simulink model "DC_grid_SCPF"  (R2023b)
settings: Solver=FixedStepAuto  StartTime=0.0  StopTime=5  FixedStep=ts  RelTol=1e-3
values from neighbouring files (symbols this model uses):
  C = 1.4e-3    (= 0.0014)    [param.m]
  Ic = 300    [param.m]
  L = 0.6e-3    (= 0.0006)    [param.m]
  Lt = 100    [param.m]
  nt = Essaim(1,index)    [ObjContr.m]    (also in param.m = 5)
  Ps_ref = 2.5e6    (= 2500000)    [param.m]
  R = 40e-3    (= 0.04)    [param.m]
  Rsh = 50e-3    (= 0.05)    [param.m]
  ts = 1e-4    (= 0.0001)    [param.m]
  Ve = 5e3    (= 5000)    [param.m]
libraries: spsCurrentMeasurementLib x3, spsSeriesRLCBranchLib x3, spsVoltageMeasurementLib x2, spsControlledCurrentSourceLib x1, spsDCVoltageSourceLib x1, spsGroundLib x1, spsControlledVoltageSourceLib x1, sps_lib x1
settings Model: Creator=user  LastModifiedBy=metta
settings DebuggingCC: AlgebraicLoopMsg=none

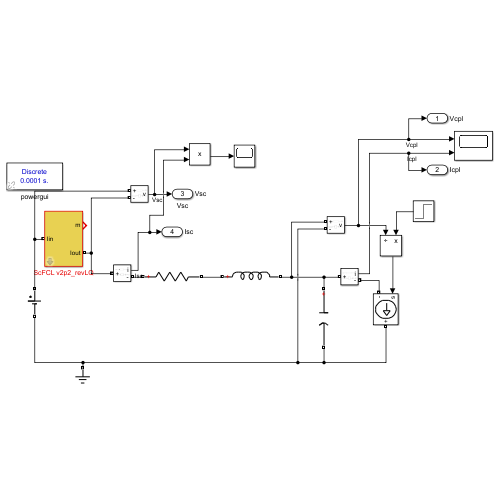
[thumbnail: Simulink's stored preview of the top-level diagram]
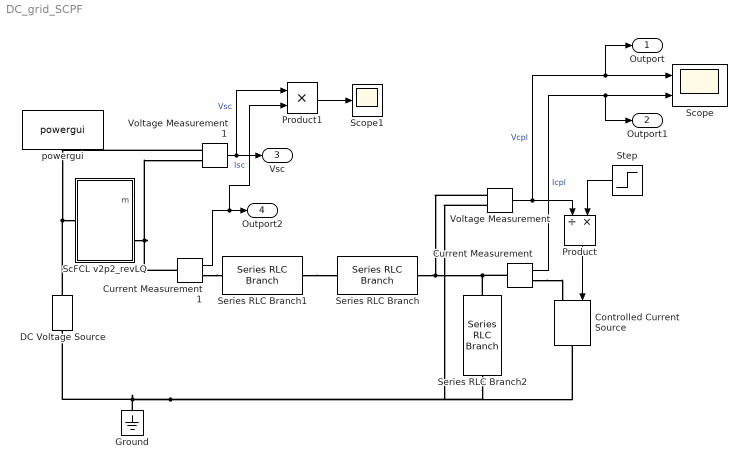
== system DC_grid_SCPF ==
  Controlled Current Source : spsControlledCurrentSourceLib/Controlled Current Source  Initialize=on  Source_Type=DC  Amplitude=0  Phase=0  Frequency=0  Measurements=None
  Current Measurement : spsCurrentMeasurementLib/Current Measurement  PhasorSimulation=off  OutputType=Complex  PSBequivalent=0
  Current Measurement1 : spsCurrentMeasurementLib/Current Measurement  PhasorSimulation=off  OutputType=Complex  PSBequivalent=0
  DC Voltage Source : spsDCVoltageSourceLib/DC Voltage Source  Amplitude=Ve  Measurements=None
  Ground : spsGroundLib/Ground  LConnTagsString=a
  Product : Product  Inputs=/*
  Product1 : Product  Inputs=**
  ScFCL v2p2_revLQ : Subsystem  mask{isScFCLWanted=on, isYBCOWanted=YBCO, Tc_ybco=92, Ic0_ybco=Ic, n0_ybco=21, tw_ybco=12, splicelessTapeLength=Lt, th_ins_ybco=32, th_stab_t=20, th_Ag_t=4, th_Sc=1, th_Hast=100, th_Ag_b=1, th_stab_b=20, Tc_bscco=110, Ic0_bscco=220, n0_bscco=15, tw_bscco=4, fSc_bscco=65, th_ins_bscco=32, th_stab_bscco=0, th_Agbscco=200, RSh=Rsh, tl=Lt, nt=nt, Tref=77, isConvectionWanted=LN2 convection curve  1}
      mask prompts: isScFCLWanted "Enable/Disable ScFCL"; isYBCOWanted "Choice of Material"; Tc_ybco "Critical temperature [K]"; Ic0_ybco "Critical current at 77 K, SF [A]"; n0_ybco "n-value at 77 K, SF"; tw_ybco "Tape width [mm]"; splicelessTapeLength "Spliceless length of tape [m]"; th_ins_ybco "Insulation"; th_stab_t "Stabilizer top"; th_Ag_t "Silver top"; th_Sc "Superconductor"; th_Hast "Hastelloy"; th_Ag_b "Silver bottom"; th_stab_b "Stabilizer bottom"; Tc_bscco "Critical temperature [K]"; Ic0_bscco "Critical current at 77 K, SF [A]"; n0_bscco "n-value at 77 K, SF"; tw_bscco "Tape width [mm]"; fSc_bscco "Percentage of superconductor"; th_ins_bscco "Insulation"; th_stab_bscco "Additional stabilizer (Cu, 304SS, ...)"; th_Agbscco "Ag-BSCCO"; RSh "Shunt resistance [Ohm]:"; tl "Length of tapes [m]:"; nt "Number of tapes in parallel"; Tref "Temperature of reference [K]"; isConvectionWanted "Cooling scheme"
      mask init:
      | if ~isScFCLWanted
      |     tl = 1e-24;
      | end
      | switch isYBCOWanted
      |     case 1 %YBCO
      |         Tc = Tc_ybco;
      |         Ic0 = Ic0_ybco;
      |         n0 = n0_ybco;
      |         tw = 1e-3*tw_ybco; %[m]
      |         th = 1e-6*[th_ins_ybco; th_stab_t; th_Ag_t; th_Sc; th_Hast; th_Ag_b; th_stab_b; th_ins_ybco]; %[m]
      |         th(th == 0) = 1e-12; % If some thickness are zeros, replace by a small value to allow a proper conditioning of the matrix of the system
      |         frac_sc = 0; % not used
      |         % Splice resistivity = ~40 nOhm-cm^2, 10 cm long splice according to:
      |         % Y. Tsui1, E. Surrey and D. Hampshire, "Soldered joints—an essential component of
      |         % demountable high temperature SC fusion magnets," Supercond. Sci. Technol. 29 (2016) 075005 (16pp).
      |         %Rj = (40e-9/(10*tw*1e-2))*ceil(tl/splicelessTapeLength);
      |         Rj = (1e-9)*ceil(tl/splicelessTapeLength);
      |         % It is important to provide a small resistance Rj to Rsc to avoid a bad
      |         % conditioning of the problem (RCOND = Nan in Matlab). It is less
      |         % articifial and more realistic than affecting an arbitrary value to Rsc.
      |     case 2 %BSCCO
      |         Tc = Tc_bscco;
      |         Ic0 = Ic0_bscco;
      |         n0 = n0_bscco;
      |         tw = 1e-3*tw_bscco;
      |         th = 1e-6*[th_ins_bscco; th_stab_bscco/2; th_Agbscco; th_stab_bscco/2; th_ins_bscco; 0; 0; 0]; % artificially increase the dimension for allowing persistent values and switching between materials
      |         th(th == 0) = 1e-12; 
      |         frac_sc = fSc_bscco/100; % prercentage
      |         Rj = 20e-9;
      |     otherwise % Do nothing yet
      |         Tc = Tc_ybco;
      |         Ic0 = Ic0_ybco;
      |         n0 = n0_ybco;
      |         tw = 1e-3*tw_ybco; %[m]
      |         th = 1e-6*[th_ins_ybco; th_stab_t; th_Ag_t; th_Sc; th_Hast; th_Ag_b; th_stab_b; th_ins_ybco]; %[m]
      |         th(th == 0) = 1e-12; % If some thickness are zeros, replace by a small value to allow a proper conditioning of the matrix of the system
      |         frac_sc = 0; % not used
      |         Rj = 20e-9;
      | end
      mask TypeOptions isYBCOWanted: YBCO | BSCCO
      mask TypeOptions isConvectionWanted: No thermal model (T=Tref) | Adiabatic | LN2 convection curve  1 | LN2 convection curve 2 | LN2 convection curve 3
      mask DialogControl MaterialContainer Prompt: Material properties
      mask DialogControl YBCOContainer Prompt: YBCO
      mask DialogControl ThicknessesYBCOContainer Prompt: Thickness of tape layers [um]
      mask DialogControl BSCCOContainer Prompt: BSCCO
      mask DialogControl ThicknessesBSCCOContainer Prompt: Thickness of tape layers [um]
      mask DialogControl ScFCLContainer Prompt: ScFCL
      mask DialogControl CoolingContainer Prompt: Cooling options
  Scope : Scope  NumInputPorts=2
  Scope1 : Scope
  Series RLC Branch : spsSeriesRLCBranchLib/Series RLC Branch  LConnTagsString=__new0  RConnTagsString=__new0  BranchType=L  Resistance=R  Inductance=L  SetiL0=off  InitialCurrent=0  Capacitance=1e-6  Setx0=off  InitialVoltage=0  Measurements=None
  Series RLC Branch1 : spsSeriesRLCBranchLib/Series RLC Branch  LConnTagsString=__new0  RConnTagsString=__new0  BranchType=R  Resistance=R  Inductance=1e-3  SetiL0=off  InitialCurrent=0  Capacitance=1e-6  Setx0=off  InitialVoltage=0  Measurements=None
  Series RLC Branch2 : spsSeriesRLCBranchLib/Series RLC Branch  LConnTagsString=__new0  RConnTagsString=__new0  BranchType=C  Resistance=R  Inductance=L  SetiL0=off  InitialCurrent=0  Capacitance=C  Setx0=off  InitialVoltage=0  Measurements=None
  Step : Step  Time=0.1  After=Ps_ref  SampleTime=0
  Voltage Measurement : spsVoltageMeasurementLib/Voltage Measurement  PhasorSimulation=off  OutputType=Complex  PSBequivalent=0
  Voltage Measurement1 : spsVoltageMeasurementLib/Voltage Measurement  PhasorSimulation=off  OutputType=Complex  PSBequivalent=0
  powergui : sps_lib/powergui  Priority=1  SimulationMode=Discrete  SampleTime=ts  frequency=60  Iterations=50  frequencyindice=0  Pbase=100e6  ErrMax=1e-4  UnitsV=kV  UnitsW=MW  buscounter=0  FunctionMessages=off  echomessages=off  EnableUseOfTLC=off  CurrentSourceSwitches=off  DisableSnubberDevices=off  DisableRonSwitches=off  DisableVfSwitches=off  DisplayEquations=off  AutomaticDiscreteSolvers=off  SolverType=Tustin/Backward Euler (TBE)  Interpol=off  ExternalGateDelay=off  methode=off  Ts=100  x0status=blocks  SPID=on  SwTol=0  HookPort=off  NonlinearTolerance=1e-4  nMaxIteration=100  ContinueOnMaxIteration=off  RestoreLinks=warning  ResistiveCurrentMeasurement=off  Frange=[0:2:500]  Ylog=off  Xlog=on  ShowGrid=off  save=off  variable=ZData  structure=0  ZoomFFT=off  StartTime=0.0  cycles=1  DisplayStyle=1  fundamental=60  FreqAxis=off  MaxFrequency=1000  frequencyindicesteady=1  RmsSteady=1  display=off
  Outport : Outport  SignalName=Vcpl
  Outport1 : Outport  Port=2  SignalName=Icpl
  Vsc : Outport  Port=3  SignalName=Vsc
  Outport2 : Outport  Port=4  SignalName=Isc
  wires:
  Product/1 -> Controlled Current Source/1
  Current Measurement/1 -> Outport1/1, Scope/2  "Icpl"
  Step/1 -> Product/2
  Voltage Measurement/1 -> Product/1, Outport/1, Scope/1  "Vcpl"
  Voltage Measurement1/1 -> Product1/1, Vsc/1  "Vsc"
  Current Measurement1/1 -> Product1/2, Outport2/1  "Isc"
  Product1/1 -> Scope1/1
  connections:
  Series RLC Branch1/RConn1 -- Series RLC Branch/LConn1
  Series RLC Branch/RConn1 -- Series RLC Branch2/LConn1 -- Current Measurement/LConn1 -- Voltage Measurement/LConn1
  Ground/LConn1 -- Series RLC Branch2/RConn1 -- Controlled Current Source/RConn1 -- Voltage Measurement/LConn2 -- DC Voltage Source/LConn1
  Current Measurement/RConn1 -- Controlled Current Source/LConn1
  DC Voltage Source/RConn1 -- Voltage Measurement1/LConn1 -- ScFCL v2p2_revLQ/LConn1
  ScFCL v2p2_revLQ/RConn1 -- Current Measurement1/LConn1 -- Voltage Measurement1/LConn2
  Current Measurement1/RConn1 -- Series RLC Branch1/LConn1

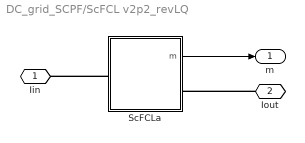
== system DC_grid_SCPF/ScFCL v2p2_revLQ ==
  ScFCLa : Subsystem
  Iin : PMIOPort  Side=Left
  Iout : PMIOPort  Port=2  Side=Right
  m : Outport
  wires:
  ScFCLa/1(m) -> m/1
  connections:
  Iout/RConn1 -- ScFCLa/RConn1
  ScFCLa/LConn1 -- Iin/RConn1

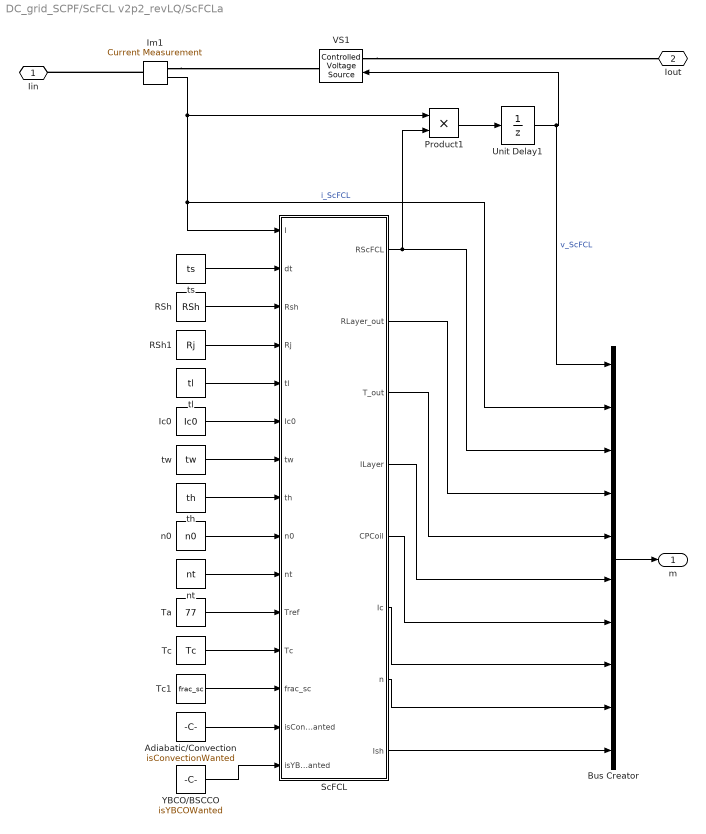
== system DC_grid_SCPF/ScFCL v2p2_revLQ/ScFCLa ==
  Adiabatic/Convection : Constant  Value=isConvectionWanted
  Bus Creator : BusCreator  Inputs=10
  Ic0 : Constant  Value=Ic0
  Im1 : spsCurrentMeasurementLib/Current Measurement  PhasorSimulation=off  OutputType=Complex  PSBequivalent=0
  Product1 : Product
  RSh : Constant  Value=RSh
  RSh1 : Constant  Value=Rj
  ScFCL : MATLAB Function  TreatAsAtomicUnit=on
  Ta : Constant  Value=77
  Tc : Constant  Value=Tc
  Tc1 : Constant  Value=frac_sc
  Unit Delay1 : UnitDelay  SampleTime=ts  HasFrameUpgradeWarning=on
  VS1 : spsControlledVoltageSourceLib/Controlled Voltage Source  Initialize=on  Source_Type=AC  Amplitude=1e-12  Phase=0  Frequency=60  Measurements=None
  YBCO/BSCCO : Constant  Value=isYBCOWanted
  n0 : Constant  Value=n0
  nt : Constant  Value=nt
  th : Constant  Value=th
  tl : Constant  Value=tl
  ts : Constant  Value=ts
  tw : Constant  Value=tw
  Iin : PMIOPort  Side=Left
  Iout : PMIOPort  Port=2  Side=Right
  m : Outport
  wires:
  Adiabatic/Convection/1 -> ScFCL/14(isConvectionWanted)
  ScFCL/1(RScFCL) -> Product1/2, Bus Creator/3
  ScFCL/2(RLayer_out) -> Bus Creator/4
  ScFCL/3(T_out) -> Bus Creator/5
  ScFCL/4(ILayer) -> Bus Creator/6
  ScFCL/5(CPCoil) -> Bus Creator/7
  ScFCL/6(Ic) -> Bus Creator/8
  ScFCL/7(n) -> Bus Creator/9
  nt/1 -> ScFCL/10(nt)
  Ta/1 -> ScFCL/11(Tref)
  n0/1 -> ScFCL/9(n0)
  th/1 -> ScFCL/8(th)
  Tc/1 -> ScFCL/12(Tc)
  Bus Creator/1 -> m/1
  Unit Delay1/1 -> Bus Creator/1, VS1/1  "v_ScFCL"
  RSh/1 -> ScFCL/3(Rsh)
  ts/1 -> ScFCL/2(dt)
  tl/1 -> ScFCL/5(tl)
  Im1/1 -> ScFCL/1(I), Bus Creator/2, Product1/1  "i_ScFCL"
  tw/1 -> ScFCL/7(tw)
  Product1/1 -> Unit Delay1/1
  Ic0/1 -> ScFCL/6(Ic0)
  YBCO/BSCCO/1 -> ScFCL/15(isYBCOWanted)
  Tc1/1 -> ScFCL/13(frac_sc)
  RSh1/1 -> ScFCL/4(Rj)
  ScFCL/8(Ish) -> Bus Creator/10
  connections:
  Im1/LConn1 -- Iin/RConn1
  Im1/RConn1 -- VS1/RConn1
  VS1/LConn1 -- Iout/RConn1

== matlab function DC_grid_SCPF/ScFCL v2p2_revLQ/ScFCLa/ScFCL ==
  data: RScFCL output; I input; RLayer_out output; T_out output; ILayer output; dt input; Rsh input; Rj input; tl input; CPCoil output; Ic0 input; Ic output; tw input; th input; n0 input; nt input; Tref input; Tc input; frac_sc input; n output; isConvectionWanted input; isYBCOWanted input; Ish output
%%% MAIN %%%
%%% Based on Jose Juan Chavez Perez's first model. Modified by Frederic Trillaud <ftrillaudp@gmail.com> & Loic Queval <loic.queval@gmail.com>.
%%% Version: 2.3 20170910
function [RScFCL, RLayer_out, T_out, ILayer, CPCoil, Ic, n, Ish] = ...
    fcn(I, dt, Rsh, Rj, tl, Ic0, tw, th, n0, nt, Tref, Tc, frac_sc, isConvectionWanted, isYBCOWanted)

%% INPUTS
% I ScFCL current [A]
% dt time step [s]
% Rsh shunt resistance [Ohm]
% Rj residual resistance due to joints (splices and connections) plus the AC base dissipation (it is useful to prevent as well a division by zero in the code) [Ohm]
% tl length of tapes [m]
% Ic0 tape critical current at 77 K, SF [A]
% tw tape width [m]
% th vector of layer thickness [m]
% n0 n-value at 77 K, SF []
% nt number of tapes in parallel []
% Tref temperature of reference [K]
% Tc critical temperature at 77 K, SF [K]
% frac_sc ? [?]
% isConvectionWanted: 1=no thermal model, 2=adiabatic, 3=curve 1, 4=curve 2, 5=curve 3 (curves of convection with LN2)
% isYBCOWanted: 1=YBCO, 2=BSCCO, 3=MgB2 unavailable

% To eliminate a layer, enter 0 in the corresponding thickness in the mask
% of the ScFCL simulink model. Automatically, instead of 0, 1e-9 will be used.
% It is necessary to allow a proper conditioning of the matrix system to solve the temperature.

%% OUPUTS
% RScFCL equivalent resistance (equivalent resistance of the fault-current limiter appearing as a resitance for the electrical circuit) [Ohm]
% RLayer_out =  Rlayer resistance of each layer [Ohm]
% T_out = T temperature of each layer [K]
% ILayer current flowing through the each layer [A]
% CPCoil Cooling power exchanged with LN2 for the nt tapes (accumulated exchanged power for the entire set of parallel superconducting tapes to be compred to DPCoil) [W]
% Ic critical current at T, SF [A]
% n n-value at T, SF []

% To do list:
% 1. Change some of the function of thermal properties: 304SS, Cu and Ag for instance to NIST functions
% 2. Add the model of the MgB2

%% Some variables
Swl = tw*tl; % Flat surface of the tape: tape width * tape length [m^2]
Shw = tw*th; % Cross-section of the tape layer [m^2]

%% Initialization
% Inputs from previous time iterations carried out in Simulink
persistent T; %temperature of each layer [K]
persistent RLayer; %resistance of each layer [Ohm]

if isempty(T)
    T = Tref*ones(length(th), 1); %initially the temperature of each layer is Tref
end
if isempty(RLayer)
    RLayer = 1e38*ones(length(th), 1); %initially the resistance of each layer is infinite
end

switch isYBCOWanted
    case 1 % YBCO
        % (1) = top insulation
        % (2) = top stabilizer
        % (3) = top silver
        % (4) = YBCO
        % (5) = Hastelloy
        % (6) = bottom silver
        % (7) = bottom stabilizer
        % (8) = bottom insulation
        
        %%% Update %%%
        
        Ic = IcVersusT(Ic0, T(4), Tc, Tref, isYBCOWanted); % [A] Critical current of the SC layer
        n = nVersusT(n0, T(4), Tref); % [] power law index
        
        %%% Current sharing %%%
        
        % Update the resistance of each layer, RLayer is a persistant variable from the previous step
        %RLayer = Resistance(T, RLayer(4)*(th(4)*tw)/tl, tl, Shw, frac_sc, isYBCOWanted); % [Ohm] Resistance of the various layers (but not the SC layer)
        RLayer = Resistance_2p3(RLayer, T, tl, Shw, frac_sc, isYBCOWanted);
        RLayer(4) = ScResistance(RLayer, Rsh, Rj, I, T(4), Ic, nt, tw, tl, th(4), n, Tc, isYBCOWanted); % [Ohm] Resistance of the SC layer
        
        % Get the current in each layer
        RScFCL = 1/(sum(nt./RLayer)+1/Rsh); % [Ohm] Equivalent resitance of the fault current limiter
        ILayer = (RScFCL./RLayer)*I; % [A] current circulating per layer
        Ish = (RScFCL/Rsh)*I; % [A] shuunt current
        
        %%% Thermal model %%%
        
        DPLayer = RLayer.*ILayer.^2; %[W] dissipated power (DP) per layer
        
        % Cooling power (CP)
        switch isConvectionWanted
            case 2 % Adiabatic
                phi = 0; % heat flux
            case 3 % LN2 convection curve 1
                [HH, phi] = HeatTransfer_1(T(1), Tref); % top
                [HH, phi] = HeatTransfer_1(T(8), Tref); % bottom
            case 4 % LN2 convection curve 2
                [HH, phi] = HeatTransfer_2(T(1), Tref);
                [HH, phi] = HeatTransfer_2(T(8), Tref);
            case 5 % LN2 convection curve 3
                [HH, phi] = HeatTransfer_3(T(1), Tref);
                [HH, phi] = HeatTransfer_3(T(8), Tref);
            otherwise % Infinite reservoir
                phi = inf;
        end
        
        % Estimation of the new temperature:
        if isConvectionWanted ~= 1 %update only if thermal model activated
            T = UpdatedTemperature(T, Swl, th, dt, DPLayer, Tref, frac_sc, isConvectionWanted, isYBCOWanted);
        end
        
    case 2 % BSCCO
        % (1) = top insulation
        % (2) = top stabilizer
        % (3) = Ag matrix
        % (4) = BSCCO
        % (5) = bottom stabilizer,
        % (6) = bottom insulation
        
        %%% Update %%%
        
        Ic = IcVersusT(Ic0, T(3), Tc, Tref, isYBCOWanted); % [A] Critical current of the SC layer
        n = nVersusT(n0, T(3), Tref); % [] power law index
        
        %%% Current sharing %%%
        
        % Update the resistance of each layer, RLayer is a persistant variable from the previous step
        %RLayer = Resistance(T, RLayer(4)*(frac_sc*th(3)*tw)/tl, tl, Shw, frac_sc, isYBCOWanted); % To be consistent with YBCO for future simplification. See the masking function for the definition of th for both YBCO and BSCCO
        RLayer = Resistance_2p3(RLayer, T, tl, Shw, frac_sc, isYBCOWanted);
        RLayer(4) = ScResistance(RLayer, Rsh, Rj, I, T(4), Ic, nt, tw, tl, th(4), n, Tc, isYBCOWanted); % [Ohm] Resistance of the SC layer
        
        % Get the current in each layer
        RScFCL = 1/(sum(nt./RLayer)+1/Rsh); % [Ohm] Equivalent resitance of the fault current limiter
        ILayer = (RScFCL./RLayer)*I; % [A] current circulating per layer
        Ish = (RScFCL/Rsh)*I; % [A] shuunt current
        
        %%% Thermal model %%%
        
        DPLayer = RLayer.*ILayer.^2; %[W] dissipated power (DP) per layer
        DPLayer(1) = DPLayer(1); % Insulation
        DPLayer(2) = DPLayer(2); % Stabilizer
        DPLayer(3) = DPLayer(3)+DPLayer(4);   % Sum of power dissipated by Ag and BSCCO
        DPLayer(4) = DPLayer(5); % stabilizer
        DPLayer(5) = DPLayer(6); % Insulation
        DPLayer(6) = DPLayer(7);
        DPLayer(7) = 0;
        DPLayer(8) = 0;
        
        % Cooling power (CP)
        switch isConvectionWanted
            case 2 % Adiabatic
                phi = 0; % heat flux
            case 3 % LN2 convection curve 1
                [HH, phi] = HeatTransfer_1(T(1), Tref); % top
                [HH, phi] = HeatTransfer_1(T(5), Tref); % bottom
            case 4 % LN2 convection curve 2
                [HH, phi] = HeatTransfer_2(T(1), Tref);
                [HH, phi] = HeatTransfer_2(T(5), Tref);
            case 5 % LN2 convection curve 3
                [HH, phi] = HeatTransfer_3(T(1), Tref);
                [HH, phi] = HeatTransfer_3(T(5), Tref);
            otherwise % Infinite reservoir
                phi = inf;
        end
        
        % Estimation of the new temperature
        if isConvectionWanted ~= 1 %update only if thermal model activated
            T = UpdatedTemperature(T, Swl, th, dt, DPLayer, Tref, frac_sc, isConvectionWanted, isYBCOWanted);
        end
        
    otherwise
        disp('MgB2 to be implemnted');
        
        %%% Update %%%
        
        Ic = 0; % [A] Critical current of the SC layer
        n = 0; % [] power law index
        
        %%% Current sharing %%%
        
        RScFCL = inf; % [Ohm] Equivalent resitance of the fault current limiter
        ILayer = zeros(length(th), 1); % [A] current circulating per layer
        Ish = 0; % [A] shuunt current
        
        %%% Thermal model %%%
        
        DPLayer = ones(length(th), 1); %[W] dissipated power (DP) per layer
        phi = inf;
        
end

CPTapet = Swl*phi;
CPTapeb = Swl*phi;
CPCoil = nt*(CPTapet+CPTapeb); % Cooling power exchanged with LN2 for the nt tapes

% For exiting the function without error and save the current values for the next time step carried out in Simulink
T_out = T;
RLayer_out = RLayer;

end


%% AUXILIARY FUNCTIONS

% Resistance per tape
function value_R = Resistance(T, rho_sc, tl, Shw, frac_sc, isYBCOWanted) % TO DELETE IF OK

switch isYBCOWanted
    case 1 % YBCO
        rho1  = 1e25; % insulation
        rho2  = rho_Cu(T(2));
        rho3  = rho_Ag(T(3));
        rho5  = rho_Hastelloy(T(5));
        rho6  = rho_Ag(T(6));
        rho7  = rho_Cu(T(7));
        rho8  = 1e25; % insulation
        rho   = [rho1; rho2; rho3; rho_sc; rho5; rho6; rho7; rho8]; %[Ohm.m]
        R = (tl*rho)./Shw;
    case 2 % BSCCO
        rho1  = 1e25; % insulation
        rho2  = rho_Cu(T(2));
        rho3 = rho_Ag(T(3))/(1-frac_sc);
        rho5  = rho_Cu(T(4));
        rho6  = 1e25; % insulation
        rho = [rho1; rho2; rho3; rho_sc; rho5; rho6; 0; 0]; %[Ohm.m]
        R1 = (tl*rho1)/Shw(1);
        R2 = (tl*rho2)/Shw(2);
        R3 = (tl*rho3)/((1-frac_sc)*Shw(3));
        R4 = (tl*rho_sc)/(frac_sc*Shw(3));
        R5 = (tl*rho5)/Shw(4);
        R6 = (tl*rho6)/Shw(5);
        % Adding large resistivity to allow a proper computation of the
        % current layers and dissipation to solve the temperature
        R = [R1; R2; R3; R4; R5; R6; 1e38; 1e38];
    otherwise
        disp('MgB2 to be implemnted');
        rho = ones(8, 1);
        R = (tl*rho)./Shw;
end

value_R = R; %[Ohm]

end

% Update resistance of the layers except SC layer
function R = Resistance_2p3(R, T, tl, Shw, frac_sc, isYBCOWanted)

switch isYBCOWanted
    case 1 % YBCO
        %R(1) %[Ohm] top insulation
        R(2)  = rho_Cu(T(2))*tl/Shw(2); %[Ohm] top stabilizer
        R(3)  = rho_Ag(T(3))*tl/Shw(3); %[Ohm] top silver
        %R(4) %[Ohm] YBCO
        R(5)  = rho_Hastelloy(T(5))*tl/Shw(5); %[Ohm] Hastelloy
        R(6)  = rho_Ag(T(6))*tl/Shw(6); %[Ohm] bottom silver
        R(7)  = rho_Cu(T(7))*tl/Shw(7); %[Ohm] bottom stabilizer
        %R(8) %[Ohm] bottom insulation
    case 2 % BSCCO
        %R(1) %[Ohm] top insulation
        R(2) = rho_Cu(T(2))*tl/Shw(2); %[Ohm] top stabilizer
        R(3) = (rho_Ag(T(3))/(1-frac_sc))*tl/((1-frac_sc)*Shw(3)); %[Ohm] Ag matrix
        %R(4) = rho_sc*tl/(frac_sc*Shw(3)); %[Ohm] BSCCO
        R(5) = rho_Cu(T(4))*tl/Shw(4); %[Ohm] bottom stabilizer
        %R(6) %[Ohm] bottom insulation
        %R(7) %[Ohm] empty
        %R(8) %[Ohm] empty
    otherwise
        disp('MgB2 to be implemnted');
end

end

% Resistance of the superconductor [Ohm]
function value_Rsc = ScResistance(Rlayer, Rsh, Rj, I, Tsc, Ic, nt, tw, tl, thsc, n, Tc, isYBCOWanted)
% I = ScFCL current
% Ic = SC layer critical current
% value_Rsc = SC layer resistance in series with Rj

if (Tsc < Tc)
    % Critical electrical field and voltage
    Ec = 1e-4;  % [V/m] (1e-6*100)
    Vc = Ec*tl; % [V]
    
    % Current sharing with Newton algorithm
    RScFCL = 1/(sum(nt./Rlayer)+1/Rsh); % [Ohm] Equivalent resitance of the fault current limiter
    Rsc0 = Rlayer(4)/nt; % [Ohm] Equivalent resitance of all the SC components making the ScFCL
    Rm = 1/(1/Rlayer(2)+1/Rlayer(3)+1/Rlayer(5)+1/Rlayer(6)+1/Rlayer(7)); % [Ohm] Equivalent resitance of all the metallic layers of 1 tape
    Req = Rm*Rsh/(nt*Rsh+Rm); % [Ohm] (Rm/nt)//Rsh
    
    %version 2.2: look for the sum of the currents of the SC layers
    %     ISc0 = (RScFCL/Rsc0)*abs(I); % Aproximation of the target current (absolute value)= sum of SC layers currents
    %     ISc = NewtonRh_2p2(abs(I), ISc0, Vc, n, nt*Ic, Req); % Get sum of SC layers currents, proper than scaling to the resistance. Otherwise, it is assumed that the changing are smooth enough to be caught from the previous time step. I do not think that it is true with a large n-value.
    %     Rsc_1 = (Vc*ISc^(n-1)/((nt*Ic)^n))*nt; % ok because keep in mind that this is Ic*=m*Ic
    
    %version 2.3: look for the current in one SC layer
    ISc0 = (RScFCL/Rsc0)*abs(I)/nt; % Aproximation of the target current (absolute value)= current of the SC layer
    ISc = NewtonRh_2p3(abs(I), ISc0, Vc, n, Ic, Req, nt); % Get current of the SC layer current, proper than scaling to the resistance. Otherwise, it is assumed that the changing are smooth enough to be caught from the previous time step. I do not think that it is true with a large n-value.
    Rsc_1 = (Vc*ISc^(n-1)/(Ic^n));
    
    switch isYBCOWanted
        case 1 % YBCO
            Rsc_2 = rho_YBCO(Tsc)*tl/(thsc*tw);
        case 2 %BSCCO
            Rsc_2 = rho_BSCCO(Tsc, Tc)*tl/(thsc*tw);
        otherwise
            Rsc_2 = rho_YBCO(Tsc)*tl/(thsc*tw);
    end
    Rsc  = min(Rsc_1, Rsc_2);
    
else % Normal state
    switch isYBCOWanted
        case 1 % YBCO
            Rsc = rho_YBCO(Tsc)*tl/(thsc*tw);
        case 2 %BSCCO
            Rsc = rho_BSCCO(Tsc, Tc)*tl/(thsc*tw);
        otherwise
            Rsc = rho_YBCO(Tsc)*tl/(thsc*tw);
    end
end

value_Rsc = Rsc+Rj; % better than putting a condition to ensure a proper conditioning of the system (avoiding division by zero). In addition, it makes sense that there should be a base dissipation and slices driving a residual resistance at the superconducting layer.

end

% Current sharing
function value_ISc = NewtonRh_2p2(I, Isc0, Vc, n, Ic, Req)

%stop conditions
maxIter = 1000;
tol = 1e-6;

%initialization
error = 1000; %initialize the error
j = 1; %initialize the iteration number
Isc = Isc0; %initial guess

while ((error > tol) && (j <= maxIter))
    f = Vc*(Isc/Ic)^n+Req*Isc-Req*I;
    df = n* Vc*Isc^(n-1)/(Ic^n)+Req;
    Isc = Isc-f/df;
    
    error = abs(f);
    j = j+1;
    if (j > maxIter)
        disp('Maximum number of iteration reached, error = %g', error);
        break
    end
end

value_ISc = Isc;

end

function value_ISc = NewtonRh_2p3(I, Isc0, Vc, n, Ic, Req, nt)

%stop conditions
maxIter = 1000;
tol = 1e-6;

%initialization
error = 1000; %initialize the error
j = 1; %initialize the iteration number
Isc = Isc0; %initial guess

while ((error > tol) && (j <= maxIter))
    f = Vc*(Isc/Ic)^n - Req*I + Req*nt*Isc;
    df = n*Vc*Isc^(n-1)/Ic^n + Req*nt;
    Isc = Isc-f/df;
    
    error = abs(f);
    j = j+1;
    if (j > maxIter)
        disp('Maximum number of iteration reached, error = %g', error);
        break
    end
end

value_ISc = Isc;

end

% Ic versus T: For the moment there is no need to change or change it. I
% like to keep a certain generality at least until the version is
% completely frozen. Matter of taste.
function value_Ic = IcVersusT(Ic0, Tsc, Tc, Tref, isYBCOWanted)

switch isYBCOWanted
    case 1 % YBCO
        Ic = Ic0*(Tc-Tsc)/(Tc-Tref);
        % I propose: value_Ic = Ic0*(Tc-Tsc)/(Tc-77);
    case 2 % BSCCO
        TTref = Tsc/Tref; % TTref = Tsc/77;
        a0 = 31.1533948715955;
        a1 = -195.759566845438;
        a2 = 588.409496514242;
        a3 = -930.754142719088;
        a4 = 793.067560549802;
        a5 = -345.73762156648;
        a6 = 60.6210777447419;
        Ic = Ic0*(a0+a1*TTref+a2*TTref^2+a3*TTref^3+a4*TTref^4+a5*TTref^5+a6*TTref^6);
    otherwise
        Ic = Ic0*(Tc-Tsc)/(Tc-Tref);
end

value_Ic = Ic;

end

% N-value versus T: see previous function
function value_n = nVersusT(n0, Tsc, Tref)
value_n = n0*Tref/Tsc;
% I propose: value_n = n0*77/Tsc;
end

% Update the Temperature of the layers from Electro-thermal equivalent:
% (C, G, CG): C(Tnew-Tol)/dt = G(Told)*Tnew+CG(Told)*Tref+Qtold, pseudo-implicit Method;
% In the simulink model ts is equal to dt, ts being the time step
function value_T = UpdatedTemperature(T, Swl, th, dt, Qt, Tref, frac_sc, isConvectionWanted, isYBCOWanted)

% Matrices of heat dissipation and thermal conductances:
C = HeatCapacity(T, Swl, th, frac_sc, isYBCOWanted); % Matrix of heat capacity
G = ThermalConductance(T, Swl, th, Tref, frac_sc, isConvectionWanted, isYBCOWanted); % matrix of thermal conductance per mid layer
CG = ConvectiveConductance(T, Swl, th, Tref, isConvectionWanted, isYBCOWanted); % matrix of thermal conductance at the boundary per tape

T = inv(C+dt*G)*(C*T+dt*(CG*Tref+Qt));
% [LOIC] if you solve C(Tnew-Tol)/dt = G(Told)*Tnew+CG(Told)*Tref+Qtold, then
% G<0 and the implicit method gives:
% I do not understand. See my notes that I sent (thermal model). G is a
% matrix. If you change the sign, you have to revert the sign into the
% definition of G. It is done this way to fit the mathematical model.
% T = inv(C-dt*G)*(C*T+dt*(CG*Tref+Qt));

value_T = T;

end

% Heat capacity [J/K]
function value_C = HeatCapacity(T, Swl, th, frac_sc, isYBCOWanted)
% Density of layer materials (kg/m^3)
Dins = 1420;     % Kapton
DAg = 10470;     % Silver
DYBCO = 6300;    % YBCO
DHast = 8900;    % Hastelloy
DCu = 8960;      % Copper
DBSCCO = 6500;  % BiSCCO
D304SS = 8000;   % 304 SS

switch isYBCOWanted
    case 1 % YBCO
        % Heat capacity per layer
        Cinst = Swl*th(1)*Dins*SpecificHeatCapacity_Kapton(T(1));      % Insulation top
        CCut = Swl*th(2)*DCu*SpecificHeatCapacity_Cu(T(2));            % Stabilizer top
        CAgt = Swl*th(3)*DAg*SpecificHeatCapacity_Ag(T(3));            % Silver top
        CYBCO = Swl*th(4)*DYBCO*SpecificHeatCapacity_YBCO(T(4));       % YBCO
        CHast = Swl*th(5)*DHast*SpecificHeatCapacity_Hastelloy(T(5));  % Hastelloy
        CAgb = Swl*th(6)*DAg*SpecificHeatCapacity_Ag(T(6));            % Silver bottom
        CCub = Swl*th(7)*DCu*SpecificHeatCapacity_Cu(T(7));            % Stabilizer bottom
        Cinsb = Swl*th(8)*Dins*SpecificHeatCapacity_Kapton(T(8));      % Insulation bottom
        C = diag([Cinst, CCut, CAgt, CYBCO, CHast, CAgb, CCub, Cinsb]);  % diagonal matrix of heat capacities
    case 2 % BSCCO
        Cinst = Swl*th(1)*Dins*SpecificHeatCapacity_Kapton(T(1));        % Insulation top
        CStabt = Swl*th(2)*DCu*SpecificHeatCapacity_Cu(T(2));            % Stabilizer top
        CBSCCO = DBSCCO*SpecificHeatCapacity_BSCCO(T(3));                % BSCCO
        CAg = DAg*SpecificHeatCapacity_Ag(T(3));                         % Silver
        CAgBSCCO = ((1-frac_sc)*CAg+frac_sc*CBSCCO)*Swl*th(3);           % Ag-BSCCO
        CStabb = Swl*th(4)*DCu*SpecificHeatCapacity_Cu(T(4));            % Stabilizer bottom
        Cinsb = Swl*th(5)*Dins*SpecificHeatCapacity_Kapton(T(5));      % Insulation bottom
        % adding 1 to get an inversible matrix inv(C+dt*G) = inv(C), det(C) diff 0
        C = diag([Cinst, CStabt, CAgBSCCO, CStabb, Cinsb, 1, 1, 1]);  % diagonal matrix of heat capacities
    otherwise
        disp('MgB2 to be impmented');
        C = ones(8, 1);
end

value_C = C;

end

% Thermal conductance [W/K]
function value_G = ThermalConductance(T, Swl, th, Tref, frac_sc, isConvectionWanted, isYBCOWanted)

% Thermal resisance by convection on LN2 (K/W);
[THRconvt, THRconvb] = ConvectiveThermalResistance(T, Swl, Tref, isConvectionWanted, isYBCOWanted);

switch isYBCOWanted
    case 1 % YBCO
        % Thermal resistance per layer (K/W):
        THRinst = th(1)/(ThermalConductivity_Kapton(T(1))*Swl);     % Insulation top
        THRCut  = th(2)/(ThermalConductivity_Cu(T(2))*Swl);         % Stabilizer top
        THRAgt  = th(3)/(ThermalConductivity_Ag(T(3))*Swl);         % Silver top
        THRYBCO = th(4)/(ThermalConductivity_YBCO(T(4))*Swl);       % YBCO
        THRHast = th(5)/(ThermalConductivity_Hastelloy(T(5))*Swl);  % Hastelloy
        THRAgb  = th(6)/(ThermalConductivity_Ag(T(6))*Swl);         % Silver bottom
        THRCub  = th(7)/(ThermalConductivity_Cu(T(7))*Swl);         % Stabilizer bottom
        THRinsb = th(8)/(ThermalConductivity_Kapton(T(8))*Swl);     % Insulation bottom
        
        % Thermal conductivity of the different mid layers (see thermal-electric analogy)
        G01 = 1/(THRconvt+THRinst/2);
        G12 = 1/(THRinst/2+THRCut/2);
        G23 = 1/(THRCut/2+THRAgt/2);
        G34 = 1/(THRAgt/2+THRYBCO/2);
        G45 = 1/(THRYBCO/2+THRHast/2);
        G56 = 1/(THRHast/2+THRAgb/2);
        G67 = 1/(THRAgb/2+THRCub/2);
        G78 = 1/(THRinsb/2+THRCub/2);
        G89 = 1/(THRconvb+THRinsb/2);
        
        % matrix of thermal conductances:
        G = -diag([G01+G12, G12+G23, G23+G34, G34+G45, G45+G56, G56+G67, G67+G78, G78+G89]); % matrix diagonal of thermal conductances
        % Coeffcients off diagonal
        G(1,2) = G12;
        G(2,1) = G12;
        G(2,3) = G23;
        G(3,2) = G23;
        G(3,4) = G34;
        G(4,3) = G34;
        G(5,4) = G45;
        G(4,5) = G45;
        G(6,5) = G56;
        G(5,6) = G56;
        G(7,6) = G67;
        G(6,7) = G67;
        G(8,7) = G78;
        G(7,8) = G78;
    case 2 % BSCCO
        % Thermal resistance per layer (K/W):
        THRinst = th(1)/(ThermalConductivity_Kapton(T(1))*Swl);                   % Insulation top
        THRStabt  = th(2)/(ThermalConductivity_Cu(T(2))*Swl);                     % Stabilizer top
        k_AgBSCCO = ThermalConductivity_Ag(T(3))/(1-frac_sc)+ThermalConductivity_BSCCO(T(3))/frac_sc;
        THRAgBSCCO = th(3)/(k_AgBSCCO*Swl);                                      % Ag-BSCCO
        THRStabb = th(4)/(ThermalConductivity_Cu(T(4))*Swl);                     % Stabilizer bottom
        THRinsb = th(5)/(ThermalConductivity_Kapton(T(5))*Swl);                   % Insulation bottom
        
        % Thermal conductivity of the different mid layers (see thermal-electric analogy)
        G01 = 1/(THRconvt+THRinst/2);
        G12 = 1/(THRinst/2+THRStabt/2);
        G23 = 1/(THRStabt/2+THRAgBSCCO/2);
        G34 = 1/(THRAgBSCCO/2+THRStabb/2);
        G45 = 1/(THRStabb/2+THRinsb/2);
        G56 = 1/(THRinsb/2+THRconvb);
        
        % matrix of thermal conductances:
        G = -diag([G01+G12, G12+G23, G23+G34, G34+G45, G45+G56, 0, 0, 0]); % matrix diagonal of thermal conductances
        % Coeffcients off diagonal
        G(1,2) = G12;
        G(2,1) = G12;
        G(2,3) = G23;
        G(3,2) = G23;
        G(3,4) = G34;
        G(4,3) = G34;
        G(5,4) = G45;
        G(4,5) = G45;
        G(6,5) = 0;
        G(5,6) = 0;
        G(7,6) = 0;
        G(6,7) = 0;
        G(8,7) = 0;
        G(7,8) = 0;
    otherwise
        disp('Mgb2 to be implemented');
        G = ones(8, 8);
end

value_G = -G;

end

% Thermal conductance at the boundary [W/K]
function value_CG = ConvectiveConductance(T, Swl, th, Tref, isConvectionWanted, isYBCOWanted)

% Thermal resisTrefnce by convection on LN2 (K/W);
[THRconvt, THRconvb] = ConvectiveThermalResistance(T, Swl, Tref, isConvectionWanted, isYBCOWanted);

switch isYBCOWanted
    case 1 % YBCO
        % Thermal resistance of top and bottom layers (K/W):
        THRinst = th(1)/(ThermalConductivity_Kapton(T(1))*Swl);     % Insulation top
        THRinsb = th(8)/(ThermalConductivity_Kapton(T(8))*Swl);     % Insulation bottom
        % Thermal conductivity at the interface with the LN2
        CGt_1  = 1/(THRconvt+THRinst/2); % top
        CGb_2  = 1/(THRinsb/2+THRconvb); % bottom
        CG = [CGt_1; 0; 0; 0; 0; 0; 0; CGb_2];
    case 2 % BSCCO
        % Thermal resistance of top and bottom layers (K/W):
        THRinst = th(1)/(ThermalConductivity_Kapton(T(1))*Swl);     % Insulation top
        THRinsb = th(5)/(ThermalConductivity_Kapton(T(5))*Swl);     % Insulation bottom
        % Thermal conductivity at the interface with the LN2
        CGt_1  = 1/(THRconvt+THRinst/2); % top
        CGb_2  = 1/(THRinsb/2+THRconvb); % bottom
        CG = [CGt_1; 0; 0; 0; CGb_2; 0; 0; 0];
    otherwise
        disp('MgB2 to be implemented');
        CG = ones(8, 1);
end

value_CG = CG;

end

% Thermal conductance at the boundary [W/K]
function [value_THRconvt, value_THRconvb] = ConvectiveThermalResistance(T, Swl, Tref, isConvectionWanted, isYBCOWanted)

switch isYBCOWanted
    case 1 % YBCO
        Tb = T(8);
    case 2 % BSCCO
        Tb = T(5);
    otherwise
        disp('Mgb2 to be implmented');
        Tb = T(1);
end

% Thermal convective resistance with LN2 (K/W);
switch isConvectionWanted
    case 2 % Adiabatic
        HHt = 0; HHb = 0; % heat transfer coefficient
    case 3 % LN2 convection curve 1
        [HHt, phit] = HeatTransfer_1(T(1), Tref); % top
        [HHb, phib] = HeatTransfer_1(Tb, Tref); % bottom
    case 4 % LN2 convection curve 2
        [HHt, phit] = HeatTransfer_2(T(1), Tref);
        [HHb, phib] = HeatTransfer_2(Tb, Tref);
    case 5 % LN2 convection curve 3
        [HHt, phit] = HeatTransfer_3(T(1), Tref);
        [HHb, phib] = HeatTransfer_3(Tb, Tref);
    otherwise % Infinite reservoir
        HHt = inf; HHb = inf;
end

THRconvt = 1/(HHt*Swl);
THRconvb = 1/(HHb*Swl);

value_THRconvt = THRconvt;
value_THRconvb = THRconvb;

end


%%% Resistivity [Ohm-m] and corresponding resistances [Ohm] %%%

% Resistivity of Silver
function rho_Ag = rho_Ag(T)
p1 = -2.082e-9; p2 = 6.17e-11;
rho_Ag = p1+p2*T; %[Ohm.m]
end

% Resistivity Copper
function rho_Cu = rho_Cu(T)
p1 = -3.06e-9; p2 = 6.841e-11;
rho_Cu = p1+p2*T; %[Ohm.m]
end

% Resistivity Hastelloy
function rho_Hast = rho_Hastelloy(T)
p1 = 1.22615e-6; p2 = 1.16923e-10;
rho_Hast = p1+p2*T; %[Ohm.m]
end

% Resistivity YBCO, normal state
function rho_YBCO = rho_YBCO(T)
p1 = -1e-3; p2 = 1e-4;
rho_YBCO = p1+p2*T; %[Ohm.m]
end

% Resistivity BSCCO, normal state
function rho_BSCCO = rho_BSCCO(T, Tc)
alfa = 0.087; p1 = 1; p2 = 0.0092;
rho_BSCCO = alfa*(p1+p2*(T-Tc));
end

% % Resistivity of 304 Stainless Steel:
% function rho_304SS = Resistivity_304SS(T)
% a1 = 4.7589144;
% a2 = 0.0099003;
% na = 0.95536674;
% rho_304SS = (a1+a2*(T^na))/(10^7); %[Ohm.m]
% end

%%% Specific heat capacity [J/kg-K] %%%%

% Dresner. Protection of a test Magnet Wound with a Ag/Bi
% Specific Heat capacity of Silver
function C_Ag = SpecificHeatCapacity_Ag(T)
a0 = 1944; a1 = 24.95; n = 0.85; mol_Ag = 107.868; debye_Ag = 220;
C_Ag = 1e3*(((a0*((T/debye_Ag)^3))^(-n)+(a1^(-n)))^(-1/n))/mol_Ag; %[J/kg-K]
end

% Specific heat capacity of Copper
function C_Cu = SpecificHeatCapacity_Cu(T)
C_Cu = 390.9-539.4*exp(-0.014*T); %[J/kg-K]
end

% Specific Heat capacity of YBCO
function C_YBCO = SpecificHeatCapacity_YBCO(T)
C_YBCO = 390*(250/T)^2*(exp(250/T)/(exp(250/T)-1)^2); %[J/kg-K]
end

% Specific Heat capacity of BSCCO
function C_BSCCO = SpecificHeatCapacity_BSCCO(T)
C_BSCCO = 421*(300/T)^2*(exp(300/T)/(exp(300/T)-1)^2);
end

% Specific Heat capacity of Hastelloy
function C_Hast = SpecificHeatCapacity_Hastelloy(T)
C_Hast = 1000*(0.19+2*(0.194*(1-exp(-T/310)))); %[J/kg-K]
end

% Specific Heat capacity of Kapton
function C_Kapton = SpecificHeatCapacity_Kapton(T)
DKapton = 1420; a0 = -1.3684; a1 = 0.65892; a2 = 2.8719; a3 = 0.42651; 
a4 = -3.0088; a5 = 1.9558; a6 = -0.51998; a7 = 0.051574;
logC = a0+a1*log10(T)+a2*((log10(T))^2)+a3*((log10(T))^3)+a4*((log10(T))^4)+a5*((log10(T))^5)+a6*((log10(T))^6)+a7*((log10(T))^7);
C_Kapton = 10^logC/DKapton; %[J/kg-K]
end

% Specific Heat capacity of 304 Stainless Steel
function C_304SS = SpecificHeatCapacity_304SS(T)
a0 = 22.0061; a1 = -127.5528; a2 = 303.647; a3 = -381.0098; a4 = 274.0328;
a5 = -112.9212; a6 = 24.7593; a7 = -2.239153;
cplog = a0+a1*log10(T)+a2*((log10(T))^2)+a3*((log10(T))^3)+a4*((log10(T))^4)+a5*((log10(T))^5)+a6*((log10(T))^6)+a7*((log10(T))^7);
C_304SS = 10^cplog; %[J/kg-K]
end


%%% Thermal conductivity [W/K-m] %%%%

% Thermal Conductivity of Silver
function k_Ag = ThermalConductivity_Ag(T)
k_Ag=420.9+(501.8*0.956^T); %[W/K-m]
end
% Thermal Conductivity of Copper
function k_Cu = ThermalConductivity_Cu(T)
k_Cu=420.7+(2076*0.965^T); %[W/K-m]
end

% Thermal Conductivity of YBCO
function k_YB = ThermalConductivity_YBCO(T)
k_YB=5; %[W/K-m]
end

% Thermal Conductivity of BSCCO
function k_BSCCO = ThermalConductivity_BSCCO(T)
k_BSCCO=2.3-0.011*T+7e-5*T^2-6.6e-8*T^3;
end

% Thermal Conductivity of Hastelloy
% Ewin, Jack. Experimental Techniques for low temperature measurements
function k_Hs = ThermalConductivity_Hastelloy(T)
a0 = 5.726708; a1 = 1.349819e-2; a2 = 3.565928e-6;
k_Hs = a0+a1*T+a2*(T^2); %[W/K-m]
end

% Thermal conductivity of Kapton
function k_Kap = ThermalConductivity_Kapton(T)
a0 = -1.99117145; a1 = -0.84948679; a2 = 1.99072759; a3 = -0.88969722; a4 = 0.12450124;
logk = a0+a1*log10(T)+a2*((log10(T))^2)+a3*((log10(T))^3)+a4*((log10(T))^4);
k_Kap = 10^logk; %[W/K-m]
end

% 304 Stainless Steel:
function k_304SS = ThermalConductivity_304SS(T)
a0 = -1.4087; a1 = 1.3982; a2 = 0.2543; a3 = -0.626; a4 = 0.2334;
a5 = 0.4256; a6 = -0.4658; a7 = 0.1650; a8 = -0.0199;
logk = a0+a1*log10(T)+a2*((log10(T))^2)+a3*((log10(T))^3)+a4*((log10(T))^4)+a5*((log10(T))^5)+a6*((log10(T))^6)+a7*((log10(T))^7)+a8*((log10(T))^8);
k_304SS = 10^logk; %[W/K-m]
end


%%% Heat transfer coefficient LN2 [W/K-m^2] %%%

%%% LN2 convection - curve 1, reference: O. Mader, "Simulationen und experimente zum stabilitatsverhalten von HTSL-bandleitern,"
%%% PhD Thesis, Karlsruher Institut fur Technologie Fakultat fur
%%% Elektrotechnik und Informationstechnik.
function qc = hc_N(DT)
if (DT<3)
    q=0.217*DT;
else
    if (DT<26.5)
        a0 = 3.8147; a1 = -2.8209; a2 = 0.72328; a3 = -0.049438; a4 = 1.325e-3; a5 = -12.773e-6; 
        q=(a0+a1*DT+a2*DT^2+a3*DT^3+a4*DT^4+a5*DT^5);
    else
        q=0.0397 +97.9e-4*DT;
    end
end
qc=q*1e4; %[W/K-m^2]
end


%%% Curve 1 (reference: Trillaud)
%Heat flux of Liquid Nitrogen (W/m^2):
function [hc, qc] = HeatTransfer_1(T, Tref)
DT = T-Tref;
v1=sqrt(2)/sqrt(pi);
p0 = 0.088;
if (DT<=0)
    q=0;
else
    if ((DT>0)&&(DT<=5))
        q=1e4*p0*DT^2;
    else
        if ((DT>5)&&(DT<=11.1))
            a0 = 0.07774; a1 = 140.461; a2 = 7.738; a3 = 12.603;
            v2=(DT-a3)/a2;
            q=1e4*(a0+v1*(a1/a2)*exp(-2*(v2^2)));
        else
            if ((DT>11.1)&&(DT<=20))
                a0=3.037; a1= 237.717; a2= 15.8477; a3= 15.272;
                v2=(DT-a3)/a2;
                q=1e4*(a0+v1*(a1/a2)*exp(-2*(v2^2)));
            else
                if ((DT>20)&&(DT<=31.05))
                    a0 = -3579.81841801;
                    a1 = 676.95993494;
                    a2 = -50.06449001;
                    a3 = 1.82057088;
                    a4 = -0.03267505;
                    a5=2.32147033e-4;
                    q=1e4*(a0+a1*DT+a2*DT^2+a3*DT^3+a4*DT^4+a5*DT^5);
                else
                    a0 = 0.343;
                    a1= 0.0106;
                    a2= -2.496e-6;
                    q=1e4*(a0+a1*DT+a2*DT^2);
                end
            end
        end
    end
end
qc=q;
if (DT == 0)
    hc = 0;
else
    hc = q/DT;
end
end



%%% LN2 convection - curve 2, reference: A. D. Berger, "Stability of SC cables with twisted stacked YBCO coated conductors,"
%%% Plasma Science and Fusion Center, Massachusetts Institute of Technology, MIT, February 2012.
function [hc, qc] = HeatTransfer_2(T, Tref)
DT = T-Tref;
if (DT<=0)
    a0 = 0; a1 = 0; a2 = 0; a3 = 0; a4 = 0; a5 = 0;
else
    if (DT<=4.6)
        a5 = 0.001680087; a4 = -0.019242022; a3 = 0.087095646;
        a2 = -0.074037883; a1 = 0.057917877; a0 = 0;
    else
        if (DT<=10)
            a5 = 0.001523743; a4 = -0.042849971; a3 = 0.443404076;
            a2 = -1.846635116; a1 = 3.046099292; a0 = 0;
        else
            if (DT<=18.9)
                a5 = 0; a4 = 0; a3 = 0.030698456; a2 = -1.696351705;
                a1 = 28.57852002; a0 = -133.0831413;
            else
                if (DT<=22.8)
                    a5 = 0; a4 = 0; a3 = -0.019815625;
                    a2 = 1.546287856; a1 = -40.11763931; a0 = 347.5715056;
                else
                    if (DT<=89.9)
                        a5 = -7.8404488e-9; a4 = 2.8840356e-6; a3 = -0.0004118;
                        a2 = 0.028566069; a1 = -0.952535697; a0 = 12.89616643;
                    else
                        a5 = -3.37683125e-13; a4 = 4.008429818e-10;
                        a3 = -1.60665804e-7; a2 = 3.053044558e-5;
                        a1 = 0.009349036; a0 = 0.240726932;
                    end
                end
            end
        end
    end
end
q=a0+a1*DT+a2*DT^2+a3*DT^3+a4*DT^4+a5*DT^5;
qc= q*1e4;
if (DT == 0)
    hc = 0;
else
    hc = qc/DT;
end
end


% %%% LN2 convection - curve 3, reference: T. Jin, J. Hong, H. Zheng, K. Tang and Z. Gan,
% %%% "Measurement of boiling heat transfer coefficient in liquid nitrogen bath by inverse heat conduction method,"
% %%% Journal of Zhejiang University Science A, vol. 10, No. 5, 2009.
function [hc, qc] = HeatTransfer_3(T, Tref)
DT = T-Tref;
if (DT <= 0)
    q = 0;
else
    if (DT <= 4)
        q = 21.945*DT;
    else
        if (DT <= 19.6)
            q = 82.74-131.22*DT+37.64*DT^2-1.13*DT^3;
        else
            if (DT <= 52)
                q = 13087.8-723.04*DT+13.48*DT^2-0.084*DT^3;
            else
                q = 125 + 0.069*DT;
            end
        end
    end
end
qc = q*DT;
hc = q;
end
